simulink model "H7_1GDL_ind"  (R2022b)
settings: Solver=VariableStepAuto  StartTime=0.0  StopTime=10  RelTol=1e-3
model workspace (MAT data in the model file):
  surfaceBlockParameters = Simulink.LookupTable
  surfaceBlockParameters.Table = Simulink.lookuptable.Table
  surfaceBlockParameters.Table.Value = [145.669360614  122.326612109  101.996418654  84.6787802495  70.3736968941  59.0811685884  50.8011953324  45.5337771261  43.2789139695  44.0366058625; 185.313749978  156.270189263  130.473313595  107.923122972  88.6196173961  72.5627968658  59.7526613816  50.1892109434  43.8724455513  40.8023652052; 237.482290208  203.298417321  172.595359476  145.373116673  121.631688913  101.371076195  84.59127852  71.2922958872  61.4741282968  55.1367757489; 296.780859506  258.017174483  222.968434498  191.634639553  164.015789646  140.111884779  119.92292495  103.44891016  90.6898404082  81.6457156957; 357.815336073  315.032338952  276.198416866  241.313569815  210.377797799  183.391100818  160.353478873  141.264931963  126.125460088  114.935063248; 415.191598113  368.94978893  326.891184779  289.01578566  255.323591572  225.814602516  200.488818491  179.346239498  162.386865537  149.610696607; 463.515523826  414.37540262  369.652616441  329.347165291  293.459049169  261.988268074  234.934822007  212.298710969  194.079934958  180.278493975; 497.392991416  445.915058223  399.088590054  356.91358691  319.39004879  286.517975694  258.297367623  234.728224576  215.810546553  201.544333555; 511.429879083  458.174633941  409.804983819  366.320928719  327.722468638  294.009603579  265.18233354  241.240658522  222.184578525  208.014093548]
  surfaceBlockParameters.Table.Dimensions = [9 10]
  surfaceBlockParameters.Table.DataType = 'auto'
  surfaceBlockParameters.Table.FieldName = 'Table_force'
  surfaceBlockParameters.Breakpoints(1) = Simulink.lookuptable.Breakpoint
  surfaceBlockParameters.Breakpoints(1).Value = [-40 -31.1 -22.2 -13.3 -4.4 4.5 13.4 22.3 31.2]
  surfaceBlockParameters.Breakpoints(1).TunableSizeName = 'N1'
  surfaceBlockParameters.Breakpoints(1).Dimensions = [1 9]
  surfaceBlockParameters.Breakpoints(1).DataType = 'auto'
  surfaceBlockParameters.Breakpoints(1).FieldName = 'BP1_current'
  surfaceBlockParameters.Breakpoints(2) = Simulink.lookuptable.Breakpoint
  surfaceBlockParameters.Breakpoints(2).Value = [0.011 0.0123 0.0136 0.0149 0.0162 0.0175 0.0188 0.0201 0.0214 0.0227]
  surfaceBlockParameters.Breakpoints(2).TunableSizeName = 'N2'
  surfaceBlockParameters.Breakpoints(2).Dimensions = [1 10]
  surfaceBlockParameters.Breakpoints(2).DataType = 'auto'
  surfaceBlockParameters.Breakpoints(2).FieldName = 'BP2_airgap'
  surfaceBlockParameters.AllowMultipleInstancesOfTypeToHaveDifferentTableBreakpointSizes = 0
  surfaceBlockParameters.SupportTunableSize = 0
  surfaceBlockParameters.StructTypeInfo = Simulink.lookuptable.StructTypeInfo
  surfaceBlockParameters.StructTypeInfo.Name = 'surfaceBlockParameters_type'
  surfaceBlockParameters.StructTypeInfo.DataScope = 'Auto'
undefined symbols (not defined in the file or in its folder): airgap, current, inductance
libraries: slpidlib x2, simulink x1
settings Model: Creator=USUARIO  LastModifiedBy=USUARIO

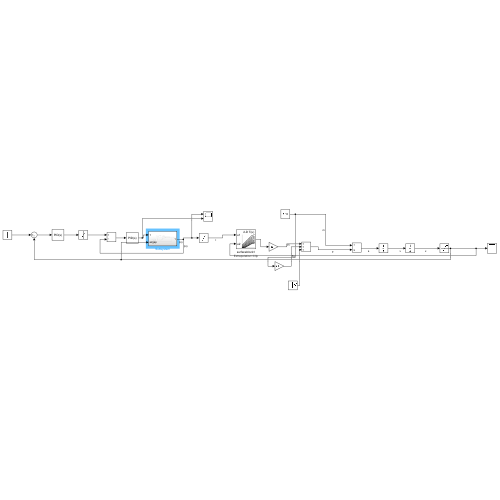
[thumbnail: Simulink's stored preview of the top-level diagram]
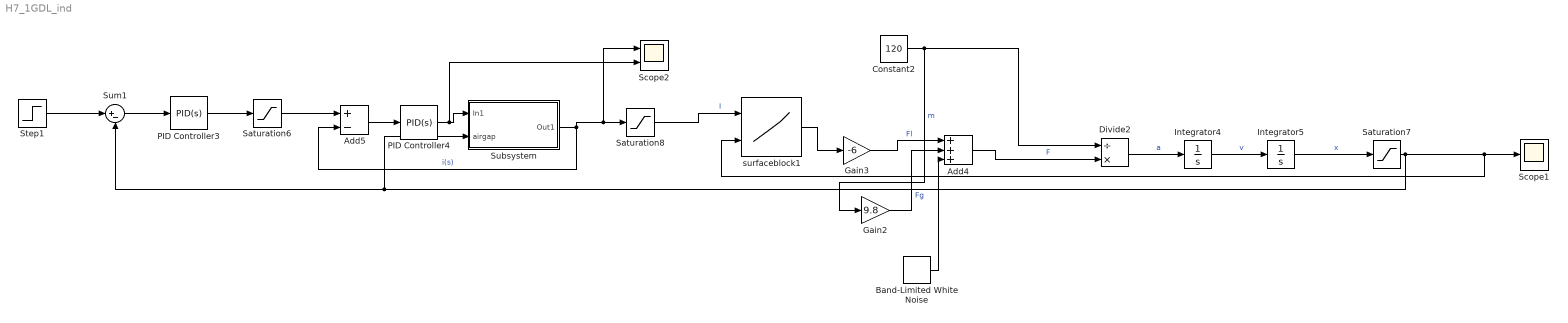
== system H7_1GDL_ind ==
  Add4 : Sum  Inputs=+++
  Add5 : Sum  Inputs=+-
  Band-Limited White Noise : simulink/Sources/Band-Limited White Noise  Cov=[2]  Ts=0.1  seed=[23341]
  Constant2 : Constant  Value=120
  Divide2 : Product  Inputs=/*
  Gain2 : Gain  Gain=9.8
  Gain3 : Gain  Gain=-6
  Integrator4 : Integrator
  Integrator5 : Integrator  InitialCondition=0.0175
  PID Controller3 : slpidlib/PID Controller  Controller=PID  Form=Parallel  TimeDomain=Continuous-time  UseExternalTs=off  SampleTime=-1  IntegratorMethod=Forward Euler  FilterMethod=Forward Euler  ControllerParametersSource=internal  P=-90039.5075843937  I=-1426732.21591299  UseKiTs=off  D=-1395.2982301274  N=1846.03168412766  UseFilter=on  TunerSelectOption=Transfer Function Based (PID Tuner App)  InitialConditionSource=internal  InitialConditionForIntegrator=0  InitialConditionForFilter=0  DifferentiatorICPrevScaledInput=0  ExternalReset=none  TrackingMode=off  Kt=1  LimitOutput=off  SatLimitsSource=internal  UpperSaturationLimit=inf  LowerSaturationLimit=-inf  LinearizeAsGain=on  AntiWindupMode=none  Kb=1  LimitIntegrator=off  UpperIntegratorSaturationLimit=inf  LowerIntegratorSaturationLimit=-inf  POutMin=[]  POutMax=[]  IOutMin=[]  IOutMax=[]  DOutMin=[]  DOutMax=[]  NOutMin=[]  NOutMax=[]  SumOutMin=[]  SumOutMax=[]  SaturationOutMin=[]  SaturationOutMax=[]  PParamMin=[]  PParamMax=[]  IParamMin=[]  IParamMax=[]  DParamMin=[]  DParamMax=[]  NParamMin=[]  NParamMax=[]  KbParamMin=[]  KbParamMax=[]  KtParamMin=[]  KtParamMax=[]  KbOutMin=[]  KbOutMax=[]  KtOutMin=[]  KtOutMax=[]  IntegratorOutMin=[]  IntegratorOutMax=[]  FilterOutMin=[]  FilterOutMax=[]  SumI1OutMin=[]  SumI1OutMax=[]  SumI2OutMin=[]  SumI2OutMax=[]  SumI3OutMin=[]  SumI3OutMax=[]  SumI4OutMin=[]  SumI4OutMax=[]  SumDOutMin=[]  SumDOutMax=[]  DifferentiatorOutMin=[]  DifferentiatorOutMax=[]  FilterDiffOutCoefMin=[]  FilterDiffOutCoefMax=[]  ReciprocalOutMin=[]  ReciprocalOutMax=[]  SumDenOutMin=[]  SumDenOutMax=[]  SumNumOutMin=[]  SumNumOutMax=[]  DivideOutMin=[]  DivideOutMax=[]  UdiffTsProdOutMin=[]  UdiffTsProdOutMax=[]  NTsProdOutMin=[]  NTsProdOutMax=[]  UintegralTsProdOutMin=[]  UintegralTsProdOutMax=[]  UngainTsProdOutMin=[]  UngainTsProdOutMax=[]  ClampingZeroOutDataTypeStr=Inherit: Inherit via back propagation  ClampingZeroOutMin=[]  ClampingZeroOutMax=[]  FilterDenConstantOutDataTypeStr=Inherit: Inherit via back propagation  FilterDenConstantOutMin=[]  FilterDenConstantOutMax=[]  PCopyOutDataTypeStr=Inherit: Inherit via back propagation  PCopyOutMin=[]  PCopyOutMax=[]  NCopyOutDataTypeStr=Inherit: Inherit via back propagation  NCopyOutMin=[]  NCopyOutMax=[]  IntegratorContinuousStateAttributes=''  IntegratorStateMustResolveToSignalObject=off  IntegratorRTWStateStorageClass=Auto  FilterContinuousStateAttributes=''  FilterStateMustResolveToSignalObject=off  FilterRTWStateStorageClass=Auto  ParallelPVariant=InternalParameters  IdealPVariant=Disabled  IVariant=InternalParameters  DVariant=InternalParameters  IntegratorVariant=Continuous  SatVariant=Disabled  AWVariant=Passthrough  PCopyVariant=Disabled  TRVariant=Disabled  FdbkBlocksVariant=Forward  IdealPFdbkVariant=Disabled  SatFdbkVariant=Disabled  DerivativeFilterVariant=ContFilter  NVariant=InternalParameters  NCopyVariant=Disabled  FilterICVariant=InternalICsFilter  IntegratorICVariant=InternalICs  ExternalResetVariant=Disabled  TRSumVariant=Passthrough  SumFdbkVariant=Disabled  SumVariant=Sum_PID  TsampFilterVariant=InternalTs  TsampNgainVariant=Passthrough  TsampIntegralVariant=Passthrough  ExternalSaturationOutDataTypeStr=Inherit: Same as second input
  PID Controller4 : slpidlib/PID Controller  Controller=PID  Form=Parallel  TimeDomain=Continuous-time  UseExternalTs=off  SampleTime=-1  IntegratorMethod=Forward Euler  FilterMethod=Forward Euler  ControllerParametersSource=internal  P=66.4403590959712  I=100871.168373079  UseKiTs=off  D=-0.000778535991956248  N=85340.1252895511  UseFilter=on  TunerSelectOption=Transfer Function Based (PID Tuner App)  InitialConditionSource=internal  InitialConditionForIntegrator=0  InitialConditionForFilter=0  DifferentiatorICPrevScaledInput=0  ExternalReset=none  TrackingMode=off  Kt=1  LimitOutput=off  SatLimitsSource=internal  UpperSaturationLimit=inf  LowerSaturationLimit=-inf  LinearizeAsGain=on  AntiWindupMode=none  Kb=1  LimitIntegrator=off  UpperIntegratorSaturationLimit=inf  LowerIntegratorSaturationLimit=-inf  POutMin=[]  POutMax=[]  IOutMin=[]  IOutMax=[]  DOutMin=[]  DOutMax=[]  NOutMin=[]  NOutMax=[]  SumOutMin=[]  SumOutMax=[]  SaturationOutMin=[]  SaturationOutMax=[]  PParamMin=[]  PParamMax=[]  IParamMin=[]  IParamMax=[]  DParamMin=[]  DParamMax=[]  NParamMin=[]  NParamMax=[]  KbParamMin=[]  KbParamMax=[]  KtParamMin=[]  KtParamMax=[]  KbOutMin=[]  KbOutMax=[]  KtOutMin=[]  KtOutMax=[]  IntegratorOutMin=[]  IntegratorOutMax=[]  FilterOutMin=[]  FilterOutMax=[]  SumI1OutMin=[]  SumI1OutMax=[]  SumI2OutMin=[]  SumI2OutMax=[]  SumI3OutMin=[]  SumI3OutMax=[]  SumI4OutMin=[]  SumI4OutMax=[]  SumDOutMin=[]  SumDOutMax=[]  DifferentiatorOutMin=[]  DifferentiatorOutMax=[]  FilterDiffOutCoefMin=[]  FilterDiffOutCoefMax=[]  ReciprocalOutMin=[]  ReciprocalOutMax=[]  SumDenOutMin=[]  SumDenOutMax=[]  SumNumOutMin=[]  SumNumOutMax=[]  DivideOutMin=[]  DivideOutMax=[]  UdiffTsProdOutMin=[]  UdiffTsProdOutMax=[]  NTsProdOutMin=[]  NTsProdOutMax=[]  UintegralTsProdOutMin=[]  UintegralTsProdOutMax=[]  UngainTsProdOutMin=[]  UngainTsProdOutMax=[]  ClampingZeroOutDataTypeStr=Inherit: Inherit via back propagation  ClampingZeroOutMin=[]  ClampingZeroOutMax=[]  FilterDenConstantOutDataTypeStr=Inherit: Inherit via back propagation  FilterDenConstantOutMin=[]  FilterDenConstantOutMax=[]  PCopyOutDataTypeStr=Inherit: Inherit via back propagation  PCopyOutMin=[]  PCopyOutMax=[]  NCopyOutDataTypeStr=Inherit: Inherit via back propagation  NCopyOutMin=[]  NCopyOutMax=[]  IntegratorContinuousStateAttributes=''  IntegratorStateMustResolveToSignalObject=off  IntegratorRTWStateStorageClass=Auto  FilterContinuousStateAttributes=''  FilterStateMustResolveToSignalObject=off  FilterRTWStateStorageClass=Auto  ParallelPVariant=InternalParameters  IdealPVariant=Disabled  IVariant=InternalParameters  DVariant=InternalParameters  IntegratorVariant=Continuous  SatVariant=Disabled  AWVariant=Passthrough  PCopyVariant=Disabled  TRVariant=Disabled  FdbkBlocksVariant=Forward  IdealPFdbkVariant=Disabled  SatFdbkVariant=Disabled  DerivativeFilterVariant=ContFilter  NVariant=InternalParameters  NCopyVariant=Disabled  FilterICVariant=InternalICsFilter  IntegratorICVariant=InternalICs  ExternalResetVariant=Disabled  TRSumVariant=Passthrough  SumFdbkVariant=Disabled  SumVariant=Sum_PID  TsampFilterVariant=InternalTs  TsampNgainVariant=Passthrough  TsampIntegralVariant=Passthrough  ExternalSaturationOutDataTypeStr=Inherit: Same as second input
  Saturation6 : Saturate  UpperLimit=40  LowerLimit=-40
  Saturation7 : Saturate  UpperLimit=0.025  LowerLimit=0.01
  Saturation8 : Saturate  UpperLimit=40  LowerLimit=-40
  Scope1 : Scope
  Scope2 : Scope  NumInputPorts=2
  Step1 : Step  Before=0.0175  After=0.0175  SampleTime=0
  Subsystem : Subsystem
  Sum1 : Sum  Inputs=|+-
  surfaceblock1 : Lookup_n-D  DataSpecification=Lookup table object  LookupTableObject=surfaceBlockParameters  BreakpointsForDimension1=[1:3]  BreakpointsForDimension2=[1:3]  ExtrapMethod=Clip  InternalRulePriority=Speed  RndMeth=Simplest
      settings: AttributesFormatString=Extrapolation=%<ExtrapMethod>  InputPortMap=u0,u1
  wires:
  Step1/1 -> Sum1/1
  Saturation6/1 -> Add5/1
  surfaceblock1/1 -> Gain3/1
  PID Controller3/1 -> Saturation6/1
  Gain2/1 -> Add4/2  "Fg"
  Integrator5/1 -> Saturation7/1  "x"
  Gain3/1 -> Add4/1  "Fl"
  Add4/1 -> Divide2/2  "F"
  PID Controller4/1 -> Scope2/2, Subsystem/1(In1)
  Add5/1 -> PID Controller4/1
  Divide2/1 -> Integrator4/1  "a"
  Constant2/1 -> Gain2/1, Divide2/1  "m"
  Integrator4/1 -> Integrator5/1  "v"
  Sum1/1 -> PID Controller3/1
  Band-Limited White Noise/1 -> Add4/3
  Saturation8/1 -> surfaceblock1/1  "I"
  Saturation7/1 -> Scope1/1, surfaceblock1/2, Sum1/2, Subsystem/2(airgap)
  Subsystem/1(Out1) -> Scope2/1, Saturation8/1, Add5/2  "i(s)"

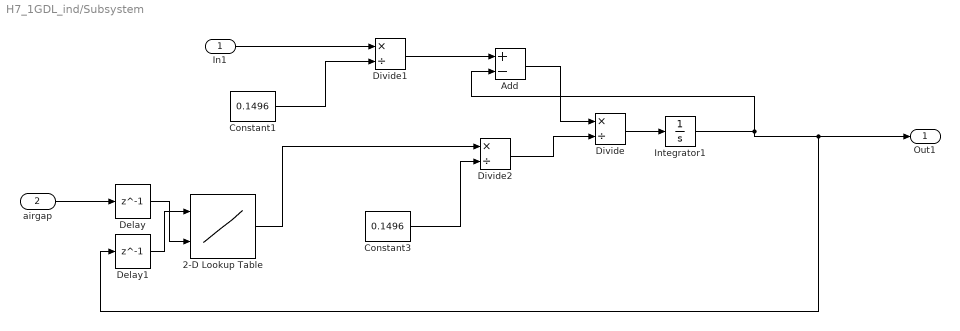
== system H7_1GDL_ind/Subsystem ==
  In1 : Inport
  airgap : Inport  Port=2
  2-D Lookup Table : Lookup_n-D  BreakpointsForDimension1=current  BreakpointsForDimension2=airgap  Table=inductance  InternalRulePriority=Speed  RndMeth=Simplest
      settings: InputPortMap=u0,u1
  Add : Sum  Inputs=+-
  Constant1 : Constant  Value=0.1496
  Constant3 : Constant  Value=0.1496
  Delay : Delay  DelayLength=1
  Delay1 : Delay  DelayLength=1
  Divide : Product  Inputs=*/
  Divide1 : Product  Inputs=*/
  Divide2 : Product  Inputs=*/
  Integrator1 : Integrator
  Out1 : Outport
  wires:
  airgap/1 -> Delay/1
  Constant1/1 -> Divide1/2
  Integrator1/1 -> Delay1/1, Out1/1, Add/2
  Divide/1 -> Integrator1/1
  In1/1 -> Divide1/1
  Divide1/1 -> Add/1
  Constant3/1 -> Divide2/2
  Divide2/1 -> Divide/2
  Add/1 -> Divide/1
  Delay/1 -> 2-D Lookup Table/2
  Delay1/1 -> 2-D Lookup Table/1
  2-D Lookup Table/1 -> Divide2/1
